simulink model "doc_ostbc32"  (R2014a)
settings: Solver=FixedStepDiscrete  SolverMode=SingleTasking  StartTime=0.0  StopTime=inf  RelTol=1e-3
PreLoadFcn:
  | EbNo = 5;
  | maxNumErrs = 100;
  | maxNumBits = 1e6;
undefined symbols (not defined in the file or in its folder): commblksprivate, Info
libraries: commchan3 x7, commdigbbndpm3 x2, commmimo x2, commrandsrc2 x1, commsink2 x1
Description:
  | OSTBC over 3x2 Rayleigh fading channel
settings Model: Creator=The MathWorks Inc.
settings DataIOCC: SignalLoggingSaveFormat=ModelDataLogs
settings OptimizationCC: InlineParams=on  ExpressionDepthLimit=2147483647
settings DebuggingCC: UnderspecifiedInitializationDetection=Classic  FcnCallInpInsideContextMsg=UseLocalSettings  StateNameClashWarn=warning  StrictBusMsg=Warning
settings GRTTargetCC: CombineOutputUpdateFcns=off  GRTInterface=on

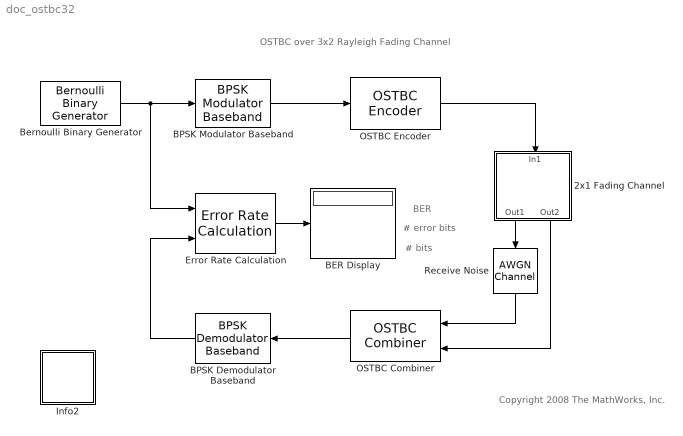
== system doc_ostbc32 ==
  note: OSTBC over 3x2 Rayleigh Fading Channel
  note: Copyright 2008 The MathWorks, Inc.
  note: BER
  note: # error bits
  note: # bits
  2x1 Fading Channel : Subsystem
      mask Display: disp('3 x 2\nFading\nChannel');
  BER Display : Display
  BPSK Demodulator Baseband : commdigbbndpm3/BPSK Demodulator Baseband  Ph=0  DecType=Hard decision  VarSource=Dialog  Variance=1  outDtype=boolean  derotateFactorWordLen=16
  BPSK Modulator Baseband : commdigbbndpm3/BPSK Modulator Baseband  Ph=0  outDtype=double  outWordLen=16  outUDDataType=sfix(16)  outFracLenMode=Best precision  outFracLen=15
  Bernoulli Binary Generator : commrandsrc2/Bernoulli Binary Generator  P=0.5  seed=61  Ts=1e-3  frameBased=on  sampPerFrame=3  orient=off  outDataType=boolean
  Error Rate Calculation : commsink2/Error Rate Calculation  N=0  st_delay=0  cp_mode=Entire frame  subframe=[]  PMode=Port  WsName=ErrorVec  RsMode2=off  stop=on  numErr=maxNumErrs  maxBits=maxNumBits
  Info2 : Subsystem  AncestorBlock=commblksprivate/Info  mask(Info){}
      settings: OpenFcn=helpview([docroot '/toolbox/comm/comm.map'], 'doc_ostbc32')
      mask Display: disp('Info')
  OSTBC Combiner : commmimo/OSTBC Combiner  numTx=3  rate=3/4  numRx=2  roundingMode=Floor  overflowMode=Wrap  crossProductWordLen=32  crossProductFracLen=16  crossSumWordLen=32  crossSumFracLen=16  egyProductWordLen=32  egyProductFracLen=16  egySumWordLen=32  egySumFracLen=16  divisionWordLen=32  divisionFracLen=16
  OSTBC Encoder : commmimo/OSTBC Encoder  numTx=3  rate=3/4  overflowMode=Wrap
  Receive Noise : commchan3/AWGN Channel  InputProcessing=Columns as channels (frame based)  seed=188  noiseMode="Signal to noise ratio  (Eb/No)"  EbNodB=EbNo - 10*log10(3)  EsNodB=5  SNRdB=EbNo - 10*log10(3)  bitsPerSym=1  Ps=2.25  Tsym=7.5e-4  variance=1
  wires:
  Bernoulli Binary Generator/1 -> BPSK Modulator Baseband/1, Error Rate Calculation/1
  BPSK Modulator Baseband/1 -> OSTBC Encoder/1
  OSTBC Encoder/1 -> 2x1 Fading Channel/1(In1)
  BPSK Demodulator Baseband/1 -> Error Rate Calculation/2
  OSTBC Combiner/1 -> BPSK Demodulator Baseband/1
  Receive Noise/1 -> OSTBC Combiner/1
  Error Rate Calculation/1 -> BER Display/1
  2x1 Fading Channel/1(Out1) -> Receive Noise/1
  2x1 Fading Channel/2(Out2) -> OSTBC Combiner/2

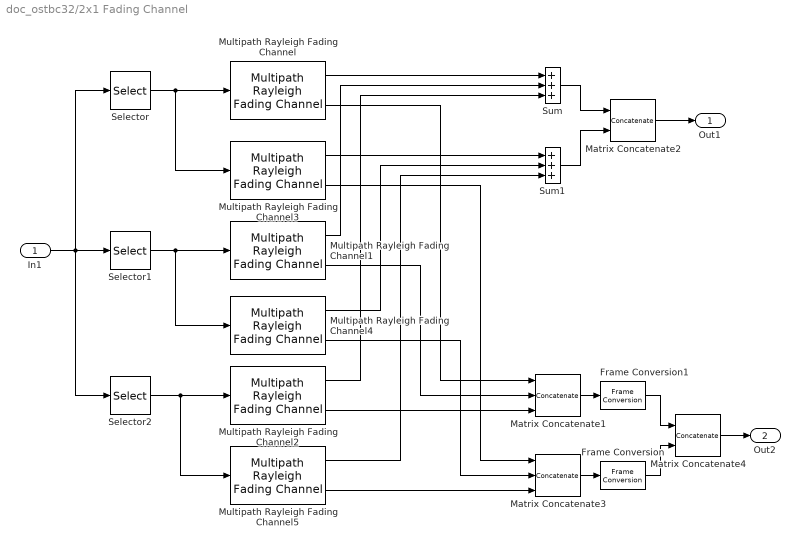
== system doc_ostbc32/2x1 Fading Channel ==
  In1 : Inport
  Frame Conversion : FrameConversion  OutFrame=Sample-based
  Frame Conversion1 : FrameConversion  OutFrame=Sample-based
  Matrix Concatenate1 : Concatenate  NumInputs=3  Mode=Multidimensional array  ConcatenateDimension=2
  Matrix Concatenate2 : Concatenate  Mode=Multidimensional array  ConcatenateDimension=2
  Matrix Concatenate3 : Concatenate  NumInputs=3  Mode=Multidimensional array  ConcatenateDimension=2
  Matrix Concatenate4 : Concatenate  Mode=Multidimensional array  ConcatenateDimension=3
  Multipath Rayleigh Fading Channel : commchan3/Multipath Rayleigh Fading Channel  maxDopplerShift=3  spectrumType=Jakes  sigmaGaussian=1/sqrt(2)  coeffRounded=[1 -1.72 0.785]  freqMinMaxRJakes=[0 1]  freqMinMaxAJakes=[0 1]  sigmaGaussian1=1/sqrt(2)  sigmaGaussian2=1/sqrt(2)  centerFreqGaussian1=0.0  centerFreqGaussian2=0.0  gainGaussian1=0.5  gainGaussian2=0.5  coeffBell=9  dopplerSpectrum=doppler.jakes  pathDelays=0  avgPathGaindB=0  normalizePathGains=on  seed=12345  enableProbe=0  openVisAtStart=off  outPathGains=on  outDelay=off
  Multipath Rayleigh Fading Channel1 : commchan3/Multipath Rayleigh Fading Channel  maxDopplerShift=3  spectrumType=Jakes  sigmaGaussian=1/sqrt(2)  coeffRounded=[1 -1.72 0.785]  freqMinMaxRJakes=[0 1]  freqMinMaxAJakes=[0 1]  sigmaGaussian1=1/sqrt(2)  sigmaGaussian2=1/sqrt(2)  centerFreqGaussian1=0.0  centerFreqGaussian2=0.0  gainGaussian1=0.5  gainGaussian2=0.5  coeffBell=9  dopplerSpectrum=doppler.jakes  pathDelays=0  avgPathGaindB=0  normalizePathGains=on  seed=24680  enableProbe=0  openVisAtStart=off  outPathGains=on  outDelay=off
  Multipath Rayleigh Fading Channel2 : commchan3/Multipath Rayleigh Fading Channel  maxDopplerShift=3  spectrumType=Jakes  sigmaGaussian=1/sqrt(2)  coeffRounded=[1 -1.72 0.785]  freqMinMaxRJakes=[0 1]  freqMinMaxAJakes=[0 1]  sigmaGaussian1=1/sqrt(2)  sigmaGaussian2=1/sqrt(2)  centerFreqGaussian1=0.0  centerFreqGaussian2=0.0  gainGaussian1=0.5  gainGaussian2=0.5  coeffBell=9  dopplerSpectrum=doppler.jakes  pathDelays=0  avgPathGaindB=0  normalizePathGains=on  seed=98765  enableProbe=0  openVisAtStart=off  outPathGains=on  outDelay=off
  Multipath Rayleigh Fading Channel3 : commchan3/Multipath Rayleigh Fading Channel  maxDopplerShift=3  spectrumType=Jakes  sigmaGaussian=1/sqrt(2)  coeffRounded=[1 -1.72 0.785]  freqMinMaxRJakes=[0 1]  freqMinMaxAJakes=[0 1]  sigmaGaussian1=1/sqrt(2)  sigmaGaussian2=1/sqrt(2)  centerFreqGaussian1=0.0  centerFreqGaussian2=0.0  gainGaussian1=0.5  gainGaussian2=0.5  coeffBell=9  dopplerSpectrum=doppler.jakes  pathDelays=0  avgPathGaindB=0  normalizePathGains=on  seed=67890  enableProbe=0  openVisAtStart=off  outPathGains=on  outDelay=off
  Multipath Rayleigh Fading Channel4 : commchan3/Multipath Rayleigh Fading Channel  maxDopplerShift=3  spectrumType=Jakes  sigmaGaussian=1/sqrt(2)  coeffRounded=[1 -1.72 0.785]  freqMinMaxRJakes=[0 1]  freqMinMaxAJakes=[0 1]  sigmaGaussian1=1/sqrt(2)  sigmaGaussian2=1/sqrt(2)  centerFreqGaussian1=0.0  centerFreqGaussian2=0.0  gainGaussian1=0.5  gainGaussian2=0.5  coeffBell=9  dopplerSpectrum=doppler.jakes  pathDelays=0  avgPathGaindB=0  normalizePathGains=on  seed=54321  enableProbe=0  openVisAtStart=off  outPathGains=on  outDelay=off
  Multipath Rayleigh Fading Channel5 : commchan3/Multipath Rayleigh Fading Channel  maxDopplerShift=3  spectrumType=Jakes  sigmaGaussian=1/sqrt(2)  coeffRounded=[1 -1.72 0.785]  freqMinMaxRJakes=[0 1]  freqMinMaxAJakes=[0 1]  sigmaGaussian1=1/sqrt(2)  sigmaGaussian2=1/sqrt(2)  centerFreqGaussian1=0.0  centerFreqGaussian2=0.0  gainGaussian1=0.5  gainGaussian2=0.5  coeffBell=9  dopplerSpectrum=doppler.jakes  pathDelays=0  avgPathGaindB=0  normalizePathGains=on  seed=13579  enableProbe=0  openVisAtStart=off  outPathGains=on  outDelay=off
  Selector : Selector  NumberOfDimensions=2  InputPortWidth=3  IndexOptions=Select all,Index vector (dialog)  Indices=-1,1
  Selector1 : Selector  NumberOfDimensions=2  InputPortWidth=3  IndexOptions=Select all,Index vector (dialog)  Indices=-1,2
  Selector2 : Selector  NumberOfDimensions=2  InputPortWidth=3  IndexOptions=Select all,Index vector (dialog)  Indices=-1,3
  Sum : Sum  Inputs=+++
  Sum1 : Sum  Inputs=+++
  Out1 : Outport
  Out2 : Outport  Port=2
  wires:
  In1/1 -> Selector1/1, Selector/1, Selector2/1
  Multipath Rayleigh Fading Channel1/1 -> Sum/2
  Multipath Rayleigh Fading Channel/1 -> Sum/1
  Multipath Rayleigh Fading Channel1/2 -> Matrix Concatenate1/2
  Multipath Rayleigh Fading Channel/2 -> Matrix Concatenate1/1
  Selector1/1 -> Multipath Rayleigh Fading Channel1/1, Multipath Rayleigh Fading Channel4/1
  Selector/1 -> Multipath Rayleigh Fading Channel/1, Multipath Rayleigh Fading Channel3/1
  Selector2/1 -> Multipath Rayleigh Fading Channel2/1, Multipath Rayleigh Fading Channel5/1
  Multipath Rayleigh Fading Channel2/1 -> Sum/3
  Multipath Rayleigh Fading Channel3/1 -> Sum1/1
  Multipath Rayleigh Fading Channel4/1 -> Sum1/2
  Multipath Rayleigh Fading Channel5/1 -> Sum1/3
  Matrix Concatenate2/1 -> Out1/1
  Sum/1 -> Matrix Concatenate2/1
  Sum1/1 -> Matrix Concatenate2/2
  Multipath Rayleigh Fading Channel2/2 -> Matrix Concatenate1/3
  Multipath Rayleigh Fading Channel3/2 -> Matrix Concatenate3/1
  Multipath Rayleigh Fading Channel4/2 -> Matrix Concatenate3/2
  Multipath Rayleigh Fading Channel5/2 -> Matrix Concatenate3/3
  Matrix Concatenate1/1 -> Frame Conversion1/1
  Matrix Concatenate3/1 -> Frame Conversion/1
  Matrix Concatenate4/1 -> Out2/1
  Frame Conversion1/1 -> Matrix Concatenate4/1
  Frame Conversion/1 -> Matrix Concatenate4/2

== system doc_ostbc32/Info2 ==
